simulink library "SimpleModeling"  (Simulink 7.7)
settings: Solver=ode45  StartTime=0.0  StopTime=10.0  RelTol=1e-3
undefined symbols (not defined in the file): pacemaker_defaults
settings Model: Creator=medcps  LastModifiedBy=iris

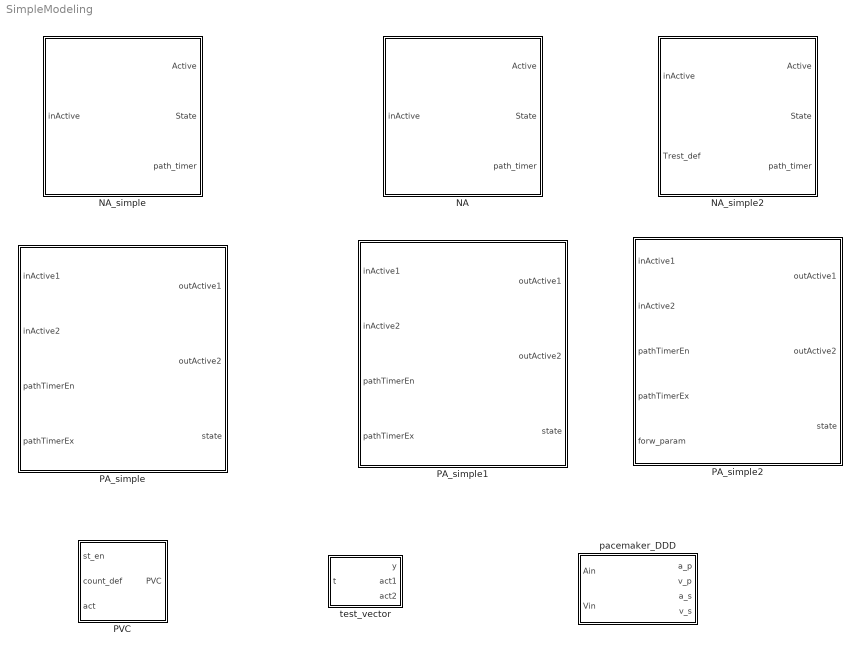
== system SimpleModeling ==
  NA : Subsystem  mask{TERP_s_m=0, TERP_defs_m=0, TRRP_s_m=0, TRRP_def_m=0, Trest_s_m=0, Trest_def_m=0, Terp_min_m=0, Terp_max_m=0}
      mask prompts: TERP_s_m "Terp Start"; TERP_defs_m "Terp Default Start"; TRRP_s_m "Trrp Start"; TRRP_def_m "Trrp Default"; Trest_s_m "Trest Start"; Trest_def_m "Trest Default"; Terp_min_m "Terp Min"; Terp_max_m "Terp Max"
  NA_simple : Subsystem  mask{TERP_s_m=0, TERP_defs_m=0, TRRP_s_m=0, TRRP_def_m=0, Trest_s_m=0, Trest_def_m=0, Terp_min_m=0, Terp_max_m=0}
      mask prompts: TERP_s_m "Terp Start"; TERP_defs_m "Terp Default Start"; TRRP_s_m "Trrp Start"; TRRP_def_m "Trrp Default"; Trest_s_m "Trest Start"; Trest_def_m "Trest Default"; Terp_min_m "Terp Min"; Terp_max_m "Terp Max"
  NA_simple2 : Subsystem  mask{TERP_s_m=0, TERP_defs_m=0, TRRP_s_m=0, TRRP_def_m=0, Trest_s_m=0, Terp_min_m=0, Terp_max_m=0}
      mask prompts: TERP_s_m "Terp Start"; TERP_defs_m "Terp Default Start"; TRRP_s_m "Trrp Start"; TRRP_def_m "Trrp Default"; Trest_s_m "Trest Start"; Terp_min_m "Terp Min"; Terp_max_m "Terp Max"
  PA_simple : Subsystem  mask{min_path_par_m=0, bck_param_m=0, forw_param_m=0}
      mask prompts: min_path_par_m "Min Path Param"; bck_param_m "Back Param"; forw_param_m "Fwd Param"
  PA_simple1 : Subsystem  mask{min_path_par_m=0, bck_param_m=0, forw_param_m=0}
      mask prompts: min_path_par_m "Min Path Param"; bck_param_m "Back Param"; forw_param_m "Fwd Param"
  PA_simple2 : Subsystem  mask{min_path_par_m=0, bck_param_m=0}
      mask prompts: min_path_par_m "Min Path Param"; bck_param_m "Back Param"
  PVC : Stateflow chart  TreatAsAtomicUnit=on
  pacemaker_DDD : Subsystem  mask{LRI_def=pacemaker_defaults(1), AVI_def=pacemaker_defaults(2), ARP_def=pacemaker_defaults(3), VRP_def=pacemaker_defaults(4), URI_def=pacemaker_defaults(5)}
      mask prompts: LRI_def "LRI default"; AVI_def "AVI default"; ARP_def "ARP default"; VRP_def "VRP default"; URI_def "URI default"
  test_vector : Stateflow chart  TreatAsAtomicUnit=on

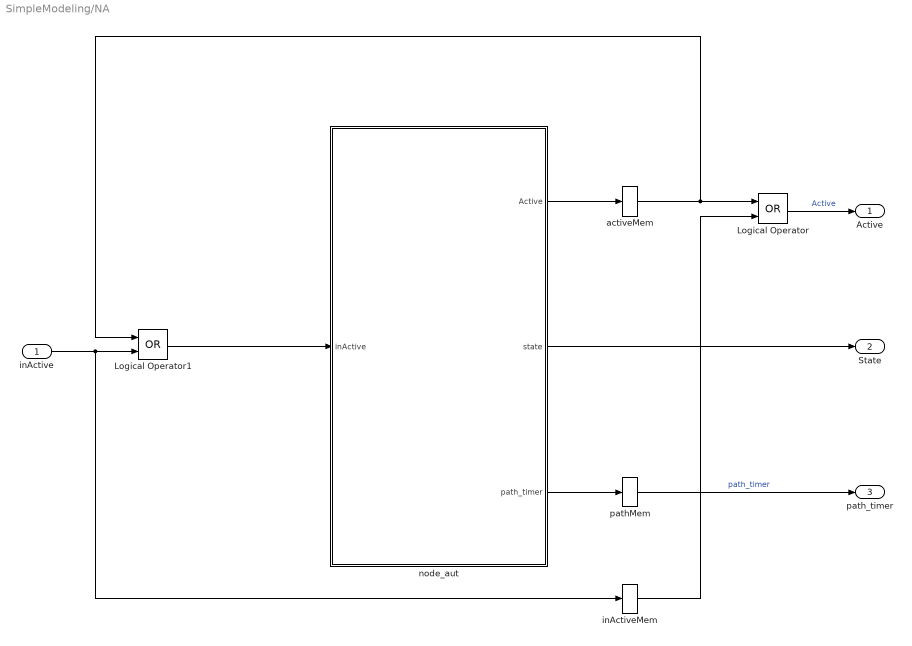
== system SimpleModeling/NA ==
  inActive : Inport
  Logical Operator : Logic  Operator=OR  AllPortsSameDT=off  OutDataTypeStr=boolean
  Logical Operator1 : Logic  Operator=OR  AllPortsSameDT=off  OutDataTypeStr=boolean
  activeMem : Memory  InheritSampleTime=on
  inActiveMem : Memory  InheritSampleTime=on
  node_aut : Stateflow chart  TreatAsAtomicUnit=on
  pathMem : Memory  InheritSampleTime=on
  Active : Outport
  State : Outport  Port=2
  path_timer : Outport  Port=3
  wires:
  node_aut/2(state) -> State/1
  pathMem/1 -> path_timer/1  "path_timer"
  node_aut/3(path_timer) -> pathMem/1
  Logical Operator/1 -> Active/1  "Active"
  inActiveMem/1 -> Logical Operator/2
  Logical Operator1/1 -> node_aut/1(inActive)
  inActive/1 -> inActiveMem/1, Logical Operator1/2
  activeMem/1 -> Logical Operator/1, Logical Operator1/1
  node_aut/1(Active) -> activeMem/1

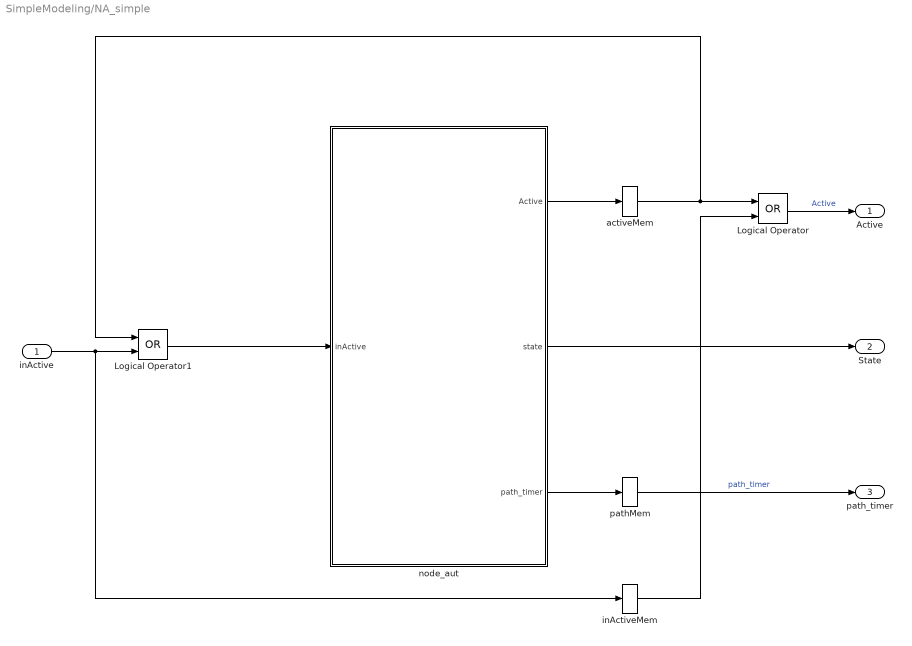
== system SimpleModeling/NA_simple ==
  inActive : Inport
  Logical Operator : Logic  Operator=OR  AllPortsSameDT=off  OutDataTypeStr=boolean
  Logical Operator1 : Logic  Operator=OR  AllPortsSameDT=off  OutDataTypeStr=boolean
  activeMem : Memory  InheritSampleTime=on
  inActiveMem : Memory  InheritSampleTime=on
  node_aut : Stateflow chart  TreatAsAtomicUnit=on
  pathMem : Memory  InheritSampleTime=on
  Active : Outport
  State : Outport  Port=2
  path_timer : Outport  Port=3
  wires:
  node_aut/1(Active) -> activeMem/1
  activeMem/1 -> Logical Operator1/1, Logical Operator/1
  inActive/1 -> Logical Operator1/2, inActiveMem/1
  Logical Operator1/1 -> node_aut/1(inActive)
  inActiveMem/1 -> Logical Operator/2
  Logical Operator/1 -> Active/1  "Active"
  node_aut/3(path_timer) -> pathMem/1
  pathMem/1 -> path_timer/1  "path_timer"
  node_aut/2(state) -> State/1

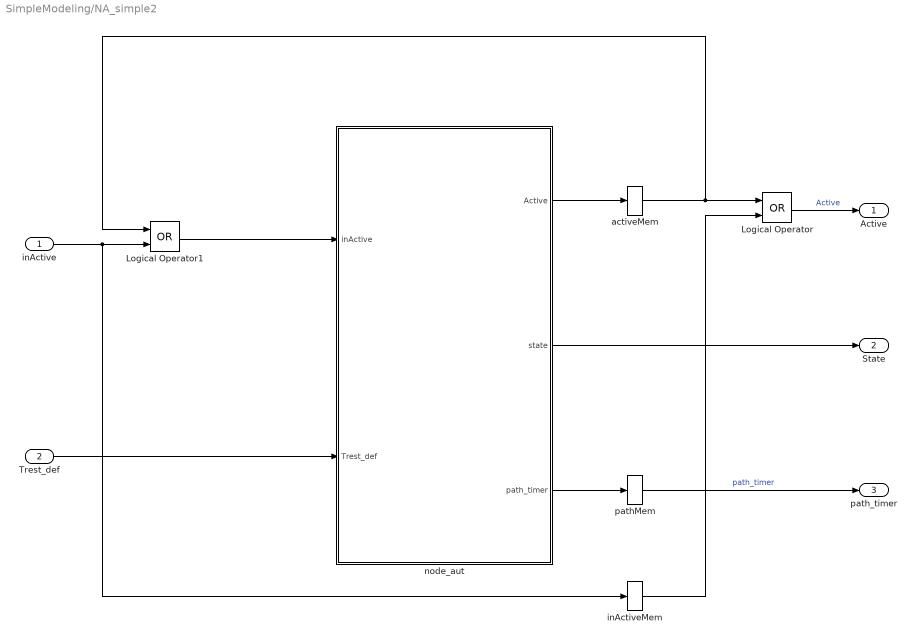
== system SimpleModeling/NA_simple2 ==
  inActive : Inport
  Trest_def : Inport  Port=2  OutDataTypeStr=uint16
  Logical Operator : Logic  Operator=OR  AllPortsSameDT=off  OutDataTypeStr=boolean
  Logical Operator1 : Logic  Operator=OR  AllPortsSameDT=off  OutDataTypeStr=boolean
  activeMem : Memory  InheritSampleTime=on
  inActiveMem : Memory  InheritSampleTime=on
  node_aut : Stateflow chart  TreatAsAtomicUnit=on
  pathMem : Memory  InheritSampleTime=on
  Active : Outport
  State : Outport  Port=2
  path_timer : Outport  Port=3
  wires:
  node_aut/2(state) -> State/1
  pathMem/1 -> path_timer/1  "path_timer"
  node_aut/3(path_timer) -> pathMem/1
  Logical Operator/1 -> Active/1  "Active"
  inActiveMem/1 -> Logical Operator/2
  Logical Operator1/1 -> node_aut/1(inActive)
  inActive/1 -> inActiveMem/1, Logical Operator1/2
  activeMem/1 -> Logical Operator/1, Logical Operator1/1
  node_aut/1(Active) -> activeMem/1
  Trest_def/1 -> node_aut/2(Trest_def)

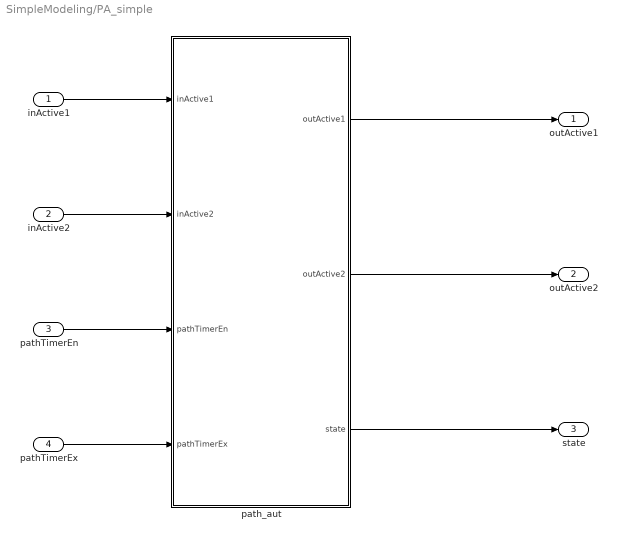
== system SimpleModeling/PA_simple ==
  inActive1 : Inport
  inActive2 : Inport  Port=2
  pathTimerEn : Inport  Port=3
  pathTimerEx : Inport  Port=4
  path_aut : Stateflow chart  TreatAsAtomicUnit=on
  outActive1 : Outport
  outActive2 : Outport  Port=2
  state : Outport  Port=3
  wires:
  inActive2/1 -> path_aut/2(inActive2)
  inActive1/1 -> path_aut/1(inActive1)
  pathTimerEn/1 -> path_aut/3(pathTimerEn)
  pathTimerEx/1 -> path_aut/4(pathTimerEx)
  path_aut/1(outActive1) -> outActive1/1
  path_aut/2(outActive2) -> outActive2/1
  path_aut/3(state) -> state/1

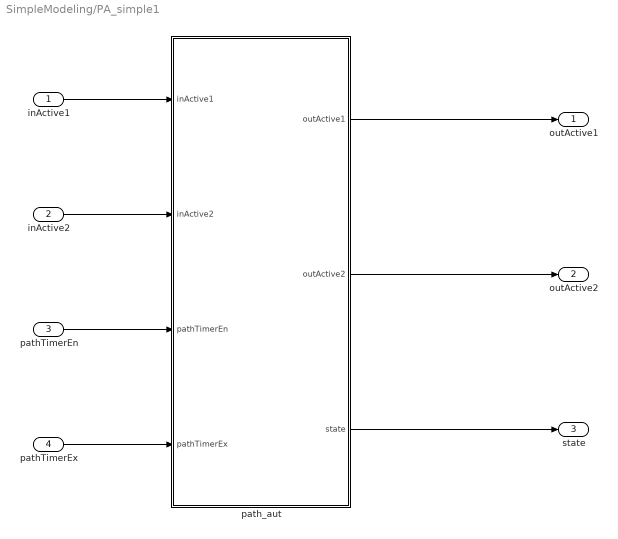
== system SimpleModeling/PA_simple1 ==
  inActive1 : Inport
  inActive2 : Inport  Port=2
  pathTimerEn : Inport  Port=3
  pathTimerEx : Inport  Port=4
  path_aut : Stateflow chart  TreatAsAtomicUnit=on
  outActive1 : Outport
  outActive2 : Outport  Port=2
  state : Outport  Port=3
  wires:
  path_aut/3(state) -> state/1
  path_aut/2(outActive2) -> outActive2/1
  path_aut/1(outActive1) -> outActive1/1
  pathTimerEx/1 -> path_aut/4(pathTimerEx)
  pathTimerEn/1 -> path_aut/3(pathTimerEn)
  inActive1/1 -> path_aut/1(inActive1)
  inActive2/1 -> path_aut/2(inActive2)

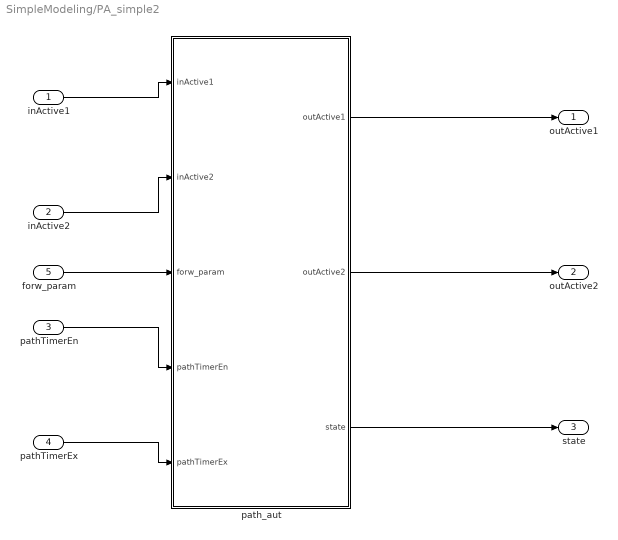
== system SimpleModeling/PA_simple2 ==
  inActive1 : Inport
  inActive2 : Inport  Port=2
  pathTimerEn : Inport  Port=3
  pathTimerEx : Inport  Port=4
  forw_param : Inport  Port=5  OutDataTypeStr=uint16
  path_aut : Stateflow chart  TreatAsAtomicUnit=on
  outActive1 : Outport
  outActive2 : Outport  Port=2
  state : Outport  Port=3
  wires:
  path_aut/3(state) -> state/1
  path_aut/2(outActive2) -> outActive2/1
  path_aut/1(outActive1) -> outActive1/1
  pathTimerEx/1 -> path_aut/5(pathTimerEx)
  pathTimerEn/1 -> path_aut/4(pathTimerEn)
  inActive1/1 -> path_aut/1(inActive1)
  inActive2/1 -> path_aut/2(inActive2)
  forw_param/1 -> path_aut/3(forw_param)

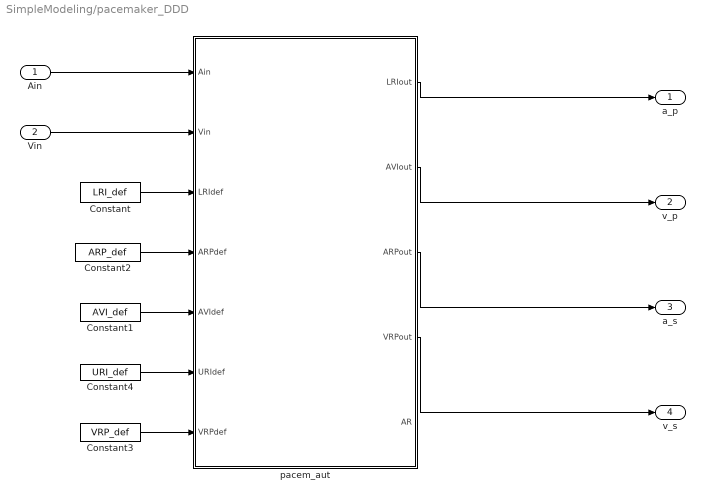
== system SimpleModeling/pacemaker_DDD ==
  Ain : Inport
  Vin : Inport  Port=2
  Constant : Constant  Value=LRI_def  OutDataTypeStr=uint16
  Constant1 : Constant  Value=AVI_def  OutDataTypeStr=uint16
  Constant2 : Constant  Value=ARP_def  OutDataTypeStr=uint16
  Constant3 : Constant  Value=VRP_def  OutDataTypeStr=uint16
  Constant4 : Constant  Value=URI_def  OutDataTypeStr=uint16
  pacem_aut : Stateflow chart  TreatAsAtomicUnit=on
  a_p : Outport
  v_p : Outport  Port=2
  a_s : Outport  Port=3
  v_s : Outport  Port=4
  wires:
  Ain/1 -> pacem_aut/1(Ain)
  Vin/1 -> pacem_aut/2(Vin)
  Constant/1 -> pacem_aut/3(LRIdef)
  Constant2/1 -> pacem_aut/4(ARPdef)
  Constant1/1 -> pacem_aut/5(AVIdef)
  Constant4/1 -> pacem_aut/6(URIdef)
  pacem_aut/1(LRIout) -> a_p/1
  pacem_aut/2(AVIout) -> v_p/1
  pacem_aut/3(ARPout) -> a_s/1
  pacem_aut/4(VRPout) -> v_s/1
  Constant3/1 -> pacem_aut/7(VRPdef)

== stateflow chart NA/node_aut ==
  settings: executeAtInitialization=1
  state NodeAutomaton
    state Rest
      du: Trest_cur = Trest_cur-1;
      du: state=1;
    state RRP
      du: TRRP_cur = TRRP_cur-1;
      du: state=3;
    state ERP
      ex: Active = 0;
      du: TERP_cur = TERP_cur-1;
      du: path_timer = 0;
      du: Active = 0;
      du: state=2;
    (default) -> Rest : {Active=0;
        | Trest_cur = Trest_s;TERP_def=TERP_defs;
        | TERP_cur = TERP_s;
        | TRRP_cur = TRRP_s;
        | path_timer = 0;}
    Rest -> ERP [order 2] : [inActive]
        | {Trest_cur = Trest_def;
        | TERP_def = Terp_max;
        | TERP_cur = Terp_max;
        | path_timer = 1;}
    ERP -> ERP [order 1] : [inActive]
        | {TERP_cur = Terp_min;
        | TERP_def = Terp_min;
        | path_timer = 3;}
    RRP -> ERP [order 1] : [inActive]
        | {ratio = TRRP_cur / TRRP_def;
        | TERP_def = Terp_min * ratio;
        | path_timer = 3;
        | TERP_cur = TERP_def;
        | TRRP_cur = TRRP_def;}
    Rest -> ERP [order 1] : [(~inActive) & (Trest_cur==0)]
        | {Trest_cur = Trest_def;
        | Active = 1;
        | path_timer = 0;}
    ERP -> RRP [order 2] : [(~inActive) & (TERP_cur==0)]
        | {TERP_cur = TERP_def;
        | path_timer = 0;}
    RRP -> Rest [order 2] : [(~inActive) & (TRRP_cur==0)]
        | {TRRP_cur = TRRP_def;
        | path_timer = 0;}
  data: TERP_cur local uint16; TRRP_cur local uint16; Trest_cur local uint16; TERP_defs constant uint16 =TERP_defs_m; TRRP_def constant uint16 =TRRP_def_m; Trest_def constant uint16 =Trest_def_m; Active output boolean; inActive input boolean; TERP_s constant uint16 =TERP_s_m; TRRP_s constant uint16 =TRRP_s_m; Trest_s constant uint16 =Trest_s_m; Terp_min constant uint16 =Terp_min_m; Terp_max constant uint16 =Terp_max_m; TERP_def local uint16; state output uint8; path_timer output uint16; ratio local uint16

== stateflow chart NA_simple/node_aut ==
  settings: executeAtInitialization=1
  state NodeAutomaton
    state Rest
      du: Trest_cur = Trest_cur-1;
      du: state=1;
    state RRP
      du: TRRP_cur = TRRP_cur-1;
      du: state=3;
    state ERP
      ex: Active = 0;
      du: TERP_cur = TERP_cur-1;
      du: path_timer = 0;
      du: Active = 0;
      du: state=2;
    (default) -> Rest : {Active=0;
        | Trest_cur = Trest_s;TERP_def=TERP_defs;
        | TERP_cur = TERP_s;
        | TRRP_cur = TRRP_s;
        | path_timer = 0;}
    Rest -> ERP [order 2] : [inActive]
        | {Trest_cur = Trest_def;
        | TERP_def = Terp_max;
        | TERP_cur = Terp_max;
        | path_timer = 1;}
    ERP -> ERP [order 1] : [inActive]
        | {TERP_cur = Terp_min;
        | TERP_def = Terp_min;
        | path_timer = 3;}
    RRP -> ERP [order 1] : [inActive]
        | {TERP_def = Terp_min;
        | path_timer = 3;
        | TERP_cur = TERP_def;
        | TRRP_cur = TRRP_def;}
    Rest -> ERP [order 1] : [(~inActive) & (Trest_cur==0)]
        | {Trest_cur = Trest_def;
        | Active = 1;
        | path_timer = 0;}
    ERP -> RRP [order 2] : [(~inActive) & (TERP_cur==0)]
        | {TERP_cur = TERP_def;
        | path_timer = 0;}
    RRP -> Rest [order 2] : [(~inActive) & (TRRP_cur==0)]
        | {TRRP_cur = TRRP_def;
        | path_timer = 0;}
  data: TERP_cur local uint16; TRRP_cur local uint16; Trest_cur local uint16; TERP_defs constant uint16 =TERP_defs_m; TRRP_def constant uint16 =TRRP_def_m; Trest_def constant uint16 =Trest_def_m; Active output boolean; inActive input boolean; TERP_s constant uint16 =TERP_s_m; TRRP_s constant uint16 =TRRP_s_m; Trest_s constant uint16 =Trest_s_m; Terp_min constant uint16 =Terp_min_m; Terp_max constant uint16 =Terp_max_m; TERP_def local uint16; state output uint8; path_timer output uint16; ratio local uint16

== stateflow chart PA_simple1/path_aut ==
  settings: executeAtInitialization=1
  state PathAutomaton [parallel]
    settings: executionOrder=3
    state Idle
      en: idle_st = 1;
      du: state=1;
    state AntegradeConduction
      du: forw_timer_cur = forw_timer_cur-1;
      du: outActive1=0;
      du: idle_st = 0;
      du: state=2;
    state Double
      du: forw_timer_cur = forw_timer_cur-1;
      du: bck_timer_cur = bck_timer_cur-1;
      du: state=5;
    state RetrogradeConduction
      du: bck_timer_cur = bck_timer_cur-1;
      du: outActive2=0;
      du: state=3;
    state Conflict
      ex: outActive2=0;
      ex: outActive1=0;
      du: state=4;
    (default) -> Idle : {outActive1=0;
        | outActive2=0;}
    Idle -> AntegradeConduction [order 1] : [inActive1]
    Idle -> RetrogradeConduction [order 2] : [(~inActive1)&&(inActive2)]
    AntegradeConduction -> Double [order 1] : [inActive2]
    Conflict -> Idle
    AntegradeConduction -> Conflict [order 2] : [forw_timer_cur==0 && (~inActive2)]
        | {forw_timer_cur=forw_timer_def;
        | outActive2=1;}
    RetrogradeConduction -> Double [order 2] : [inActive1]
    RetrogradeConduction -> Conflict [order 1] : [bck_timer_cur==0 && (~inActive1)]
        | {bck_timer_cur=bck_timer_def;
        | outActive1=1;}
    Double -> AntegradeConduction [order 1] : [bck_timer_cur==0]
        | {bck_timer_cur=bck_timer_def;
        | outActive1=1;}
    Double -> RetrogradeConduction [order 3] : [forw_timer_cur==0]
        | {forw_timer_cur=forw_timer_def;
        | outActive2=1;}
    Double -> Conflict [order 2] : [(forw_timer_cur != 0) && (bck_timer_cur != 0)]
        | {forw_timer_cur=forw_timer_def;
        | bck_timer_cur=bck_timer_def;}
  state UpdateForward [parallel]
    settings: executionOrder=1
    state Update
    UpdateForward.Update -> UpdateForward.Update [order 1] : [(pathTimerEn > 0) && (idle_st)]
        | {forw_timer_def = forw_param * pathTimerEn;
        |  forw_timer_cur = forw_timer_def;}
    UpdateForward.Update -> UpdateForward.Update [order 2] : [(pathTimerEn > 0) && (~idle_st)]
        | {forw_timer_def = forw_param * pathTimerEn;}
  state UpdateBackward [parallel]
    settings: executionOrder=2
    state Update
    UpdateBackward.Update -> UpdateBackward.Update [order 1] : [(pathTimerEx > 0) && (idle_st)]
        | {bck_timer_def = bck_param * pathTimerEx;
        |  bck_timer_cur = bck_timer_def;}
    UpdateBackward.Update -> UpdateBackward.Update [order 2] : [(pathTimerEx > 0) && (~idle_st)]
        | {bck_timer_def = bck_param * pathTimerEx;}
  data: forw_timer_cur local uint16; bck_timer_cur local uint16; outActive1 output boolean; inActive1 input boolean; inActive2 input boolean; outActive2 output boolean; min_path_par constant uint16 =min_path_par_m; bck_timer_def local uint16; forw_timer_def local uint16; bck_param constant uint16 =bck_param_m; forw_param constant uint16 =forw_param_m; idle_st local boolean; state output uint8; pathTimerEn input uint16; pathTimerEx input uint16

== stateflow chart NA_simple2/node_aut ==
  settings: executeAtInitialization=1
  state NodeAutomaton
    state Rest
      du: Trest_cur = Trest_cur-1;
      du: state=1;
    state RRP
      du: TRRP_cur = TRRP_cur-1;
      du: state=3;
    state ERP
      ex: Active = 0;
      du: TERP_cur = TERP_cur-1;
      du: path_timer = 0;
      du: Active = 0;
      du: state=2;
    (default) -> Rest : {Active=0;
        | Trest_cur = Trest_s;TERP_def=TERP_defs;
        | TERP_cur = TERP_s;
        | TRRP_cur = TRRP_s;
        | path_timer = 0;}
    Rest -> ERP [order 2] : [inActive]
        | {Trest_cur = Trest_def;
        | TERP_def = Terp_max;
        | TERP_cur = Terp_max;
        | path_timer = 1;}
    ERP -> ERP [order 1] : [inActive]
        | {TERP_cur = Terp_min;
        | TERP_def = Terp_min;
        | path_timer = 3;}
    RRP -> ERP [order 1] : [inActive]
        | {TERP_def = Terp_min;
        | path_timer = 3;
        | TERP_cur = TERP_def;
        | TRRP_cur = TRRP_def;}
    Rest -> ERP [order 1] : [(~inActive) & (Trest_cur==0)]
        | {Trest_cur = Trest_def;
        | Active = 1;
        | path_timer = 0;}
    ERP -> RRP [order 2] : [(~inActive) & (TERP_cur==0)]
        | {TERP_cur = TERP_def;
        | path_timer = 0;}
    RRP -> Rest [order 2] : [(~inActive) & (TRRP_cur==0)]
        | {TRRP_cur = TRRP_def;
        | path_timer = 0;}
  data: TERP_cur local uint16; TRRP_cur local uint16; Trest_cur local uint16; TRRP_def constant uint16 =TRRP_def_m; Active output boolean; inActive input boolean; Trest_def input uint16 =Trest_def_m; TERP_defs constant uint16 =TERP_defs_m; TERP_s constant uint16 =TERP_s_m; TRRP_s constant uint16 =TRRP_s_m; Trest_s constant uint16 =Trest_s_m; Terp_min constant uint16 =Terp_min_m; Terp_max constant uint16 =Terp_max_m; TERP_def local uint16; state output uint8; path_timer output uint16; ratio local uint16

== stateflow chart PA_simple2/path_aut ==
  settings: executeAtInitialization=1
  state PathAutomaton [parallel]
    settings: executionOrder=3
    state Idle
      en: idle_st = 1;
      du: state=1;
    state AntegradeConduction
      du: forw_timer_cur = forw_timer_cur-1;
      du: outActive1=0;
      du: idle_st = 0;
      du: state=2;
    state Double
      du: forw_timer_cur = forw_timer_cur-1;
      du: bck_timer_cur = bck_timer_cur-1;
      du: state=5;
    state RetrogradeConduction
      du: bck_timer_cur = bck_timer_cur-1;
      du: outActive2=0;
      du: state=3;
    state Conflict
      ex: outActive2=0;
      ex: outActive1=0;
      du: state=4;
    (default) -> Idle : {outActive1=0;
        | outActive2=0;}
    Idle -> AntegradeConduction [order 1] : [inActive1]
    Idle -> RetrogradeConduction [order 2] : [(~inActive1)&&(inActive2)]
    AntegradeConduction -> Double [order 1] : [inActive2]
    Conflict -> Idle
    AntegradeConduction -> Conflict [order 2] : [forw_timer_cur==0 && (~inActive2)]
        | {forw_timer_cur=forw_timer_def;
        | outActive2=1;}
    RetrogradeConduction -> Double [order 2] : [inActive1]
    RetrogradeConduction -> Conflict [order 1] : [bck_timer_cur==0 && (~inActive1)]
        | {bck_timer_cur=bck_timer_def;
        | outActive1=1;}
    Double -> AntegradeConduction [order 1] : [bck_timer_cur==0]
        | {bck_timer_cur=bck_timer_def;
        | outActive1=1;}
    Double -> RetrogradeConduction [order 3] : [forw_timer_cur==0]
        | {forw_timer_cur=forw_timer_def;
        | outActive2=1;}
    Double -> Conflict [order 2] : [(forw_timer_cur != 0) && (bck_timer_cur != 0)]
        | {forw_timer_cur=forw_timer_def;
        | bck_timer_cur=bck_timer_def;}
  state UpdateForward [parallel]
    settings: executionOrder=1
    state Update
    UpdateForward.Update -> UpdateForward.Update [order 1] : [(pathTimerEn > 0) && (idle_st)]
        | {forw_timer_def = forw_param * pathTimerEn;
        |  forw_timer_cur = forw_timer_def;}
    UpdateForward.Update -> UpdateForward.Update [order 2] : [(pathTimerEn > 0) && (~idle_st)]
        | {forw_timer_def = forw_param * pathTimerEn;}
  state UpdateBackward [parallel]
    settings: executionOrder=2
    state Update
    UpdateBackward.Update -> UpdateBackward.Update [order 1] : [(pathTimerEx > 0) && (idle_st)]
        | {bck_timer_def = bck_param * pathTimerEx;
        |  bck_timer_cur = bck_timer_def;}
    UpdateBackward.Update -> UpdateBackward.Update [order 2] : [(pathTimerEx > 0) && (~idle_st)]
        | {bck_timer_def = bck_param * pathTimerEx;}
  data: forw_timer_cur local uint16; bck_timer_cur local uint16; outActive1 output boolean; inActive1 input boolean; inActive2 input boolean; outActive2 output boolean; min_path_par constant uint16 =min_path_par_m; bck_timer_def local uint16; forw_timer_def local uint16; bck_param constant uint16 =bck_param_m; forw_param input uint16 =forw_param_m; idle_st local boolean; state output uint8; pathTimerEn input uint16; pathTimerEx input uint16

== stateflow chart pacemaker_DDD/pacem_aut ==
  state pacemakerDDD
    state LRI [parallel]
      settings: executionOrder=1
      state LRI
        du: LRIcur = LRIcur-1;
        du: LRIout = 0;
      pacemakerDDD.LRI.LRI -> pacemakerDDD.LRI.LRI [order 2] : [(LRIcur==AVIdef)&&(AVIst==1)]{LRIout=1;LRIcur = LRIcur-1;}
      (default) -> pacemakerDDD.LRI.LRI : {LRIcur=LRIdef;
          | LRIout=0;}
      pacemakerDDD.LRI.LRI -> pacemakerDDD.LRI.LRI [order 1] : [(LRIcur==0)||AVIout || VRPout]
          | {LRIcur=LRIdef; LRIout=0;}
    state AVI [parallel]
      settings: executionOrder=2
      state st1
        du: AVIout=0;
        ex: AVIout=0;
        en: AVIcur=AVIdef;
        en: AVIst = 1;
      state st2
        du: AVIcur = AVIcur-1;
        du: AVIout = 0;
      (default) -> st1 : {AVIout = 0;}
      st1 -> st2 : [LRIout||ARPout]
          | {AVIst=0;}
      st2 -> st1 [order 1] : [VRPout]{AVIout=0;}
      st2 -> st1 [order 2] : [(AVIcur<=0)&&(URIst==1)]{AVIout = 1;}
    state PVARP [parallel]
      settings: executionOrder=3
      state ARPs1
        du: ARPout=0;
      state ARPs2
        du: ARPcur = ARPcur-1;
        du: ARPout=0;
        du: AR=0;
      (default) -> ARPs1 : {ARPout=0;
          | ARPcur=ARPdef;}
      ARPs1 -> ARPs1 [order 1] : [Ain&&(AVIst==1)&&(~AVIout)&&(~VRPout)]
          | {ARPout=1;}
      ARPs1 -> ARPs2 [order 2] : [AVIout||VRPout]
          | {ARPout=0;}
      ARPs2 -> ARPs1 [order 1] : [ARPcur == 0]{ARPcur =ARPdef;}
      ARPs2 -> ARPs2 [order 2] : [Ain]
          | {AR=1;}
    state VRP [parallel]
      settings: executionOrder=4
      state VRPst2
        du: VRPcur = VRPcur-1;
        du: VRPout = 0;
      state VRPst1
        en: VRPcur = VRPdef;
      (default) -> VRPst1 : {VRPout=0;}
      VRPst1 -> VRPst2 [order 1] : [Vin]
          | {VRPout=Vin;}
      VRPst2 -> VRPst1 : [VRPcur == 0]{VRPout=0;}
      VRPst1 -> VRPst2 [order 2] : [AVIout]
          | {}
    state URI [parallel]
      settings: executionOrder=5
      state URIst1
        en: URIst=1;
        en: URIcur = URIdef;
      state URIst2
        du: URIcur = URIcur-1;
      (default) -> URIst1
      URIst1 -> URIst2 : [AVIout || VRPout]
          | {URIst = 0;}
      URIst2 -> URIst1 [order 1] : [(URIcur==0)&&(AVIcur<0)]
          | {AVIout = 1;AVIcur=AVIdef;}
      URIst2 -> URIst1 [order 2] : [URIcur==0]
  note: - Race condition?
  data: LRIcur local uint16; LRIout output boolean; Ain input boolean; AVIout output boolean; ARPout output boolean; VRPout output boolean; Vin input boolean; AVIcur local int16; ARPcur local uint16; VRPcur local uint16; URIcur local uint16; LRIdef input uint16; ARPdef input uint16; AVIdef input uint16; URIdef input uint16; AVIst local boolean; URIst local boolean; VRPdef input uint16; AR output double

== matlab function test_vector ==
  data: t input double; y output double; act1 output double; act2 output double
function [y,act1,act2] = fcn(t)
%#eml
y=1;
act1=0;
act2=0;
%    if t<2000
%        y=1;
%    end
%    if t<5000 && t>=2000
%        y=2;
%    end
%    if t<10000 && t>=5000
%        y=3;
%    end
   
%    if t==1000
%        act2=1;
%    end
%    
%    if t==4000
%        act1=1;
%    end
%    if t==8000
%        act2=1;
%    end

== stateflow chart PVC ==
  settings: executeAtInitialization=1
  state Wait
    du: PVC=0;
  state Count
    du:PVC=0;
    du: count=count-1;
  state start
    du: PVC=0;
  start -> Count : [act==1]
      | {count=count_def;}
  Count -> Wait : [count==0]
      | {PVC=1;}
  (default) -> Wait
  Wait -> start : [st_en==1]
      | {}
  data: st_en input boolean; count_def input uint16; act input boolean; PVC output boolean; count local uint16

== stateflow chart PA_simple/path_aut ==
  settings: executeAtInitialization=1
  state PathAutomaton [parallel]
    settings: executionOrder=3
    state Idle
      en: idle_st = 1;
      du: state=1;
    state AntegradeConduction
      du: forw_timer_cur = forw_timer_cur-1;
      du: outActive1=0;
      du: idle_st = 0;
      du: state=2;
    state Double
      du: forw_timer_cur = forw_timer_cur-1;
      du: bck_timer_cur = bck_timer_cur-1;
      du: state=5;
    state RetrogradeConduction
      du: bck_timer_cur = bck_timer_cur-1;
      du: outActive2=0;
      du: state=3;
    state Conflict
      ex: outActive2=0;
      ex: outActive1=0;
      du: state=4;
    (default) -> Idle : {outActive1=0;
        | outActive2=0;}
    Idle -> AntegradeConduction [order 1] : [inActive1]
    Idle -> RetrogradeConduction [order 2] : [(~inActive1)&&(inActive2)]
    AntegradeConduction -> Double [order 1] : [inActive2]
    Conflict -> Idle
    AntegradeConduction -> Conflict [order 2] : [forw_timer_cur==0 && (~inActive2)]
        | {forw_timer_cur=forw_timer_def;
        | outActive2=1;}
    RetrogradeConduction -> Double [order 2] : [inActive1]
    RetrogradeConduction -> Conflict [order 1] : [bck_timer_cur==0 && (~inActive1)]
        | {bck_timer_cur=bck_timer_def;
        | outActive1=1;}
    Double -> AntegradeConduction [order 1] : [bck_timer_cur==0]
        | {bck_timer_cur=bck_timer_def;
        | outActive1=1;}
    Double -> RetrogradeConduction [order 3] : [forw_timer_cur==0]
        | {forw_timer_cur=forw_timer_def;
        | outActive2=1;}
    Double -> Conflict [order 2] : [(forw_timer_cur != 0) && (bck_timer_cur != 0)]
        | {forw_timer_cur=forw_timer_def;
        | bck_timer_cur=bck_timer_def;}
  state UpdateForward [parallel]
    settings: executionOrder=1
    state Update
    UpdateForward.Update -> UpdateForward.Update [order 1] : [(pathTimerEn > 0) && (idle_st)]
        | {forw_timer_def = forw_param * pathTimerEn;
        |  forw_timer_cur = forw_timer_def;}
    UpdateForward.Update -> UpdateForward.Update [order 2] : [(pathTimerEn > 0) && (~idle_st)]
        | {forw_timer_def = forw_param * pathTimerEn;}
  state UpdateBackward [parallel]
    settings: executionOrder=2
    state Update
    UpdateBackward.Update -> UpdateBackward.Update [order 1] : [(pathTimerEx > 0) && (idle_st)]
        | {bck_timer_def = bck_param * pathTimerEx;
        |  bck_timer_cur = bck_timer_def;}
    UpdateBackward.Update -> UpdateBackward.Update [order 2] : [(pathTimerEx > 0) && (~idle_st)]
        | {bck_timer_def = bck_param * pathTimerEx;}
  data: forw_timer_cur local uint16; bck_timer_cur local uint16; outActive1 output boolean; inActive1 input boolean; inActive2 input boolean; outActive2 output boolean; min_path_par constant uint16 =min_path_par_m; bck_timer_def local uint16; forw_timer_def local uint16; bck_param constant uint16 =bck_param_m; forw_param constant uint16 =forw_param_m; idle_st local boolean; state output uint8; pathTimerEn input uint16; pathTimerEx input uint16
